simulink model "flexcan_encrypted_slave_s32k14x"  (Simulink 9.0)
settings: Solver=FixedStepDiscrete  StartTime=0.0  StopTime=10.0  FixedStep=0.1  RelTol=1e-3  EnableMultiTasking=on
PreLoadFcn:
  | mbd_s32k_examples_preload_cbk;
InitFcn:
  | mbd_s32k_consistency_checks(bdroot(gcs));
undefined symbols (not defined in the file): LQFP, Request, slave_receive_can_data, slave_send_can_data
libraries: mbd_s32k1xx_ec_toolbox x41, simulink x4
Description:
  | This model shows the usage of the FlexCAN module configured to use Flexible Data Rate and the CSEc module from the S32K14x MCUs.
  | 
  | The application will wait for frames to be received on the configured message buffer or for an event raised by pressing one of the two buttons, SW2 and SW3, which will trigger a frame send to the recipient.
  | On button SW3, the recipient toggles Red LED.
  | On button SW2, the recipient toggles Green LED.
  | 
  | The frames are sent in plain text by default, but the encrypted mode can be enabled by holding one of the buttons pressed and pressing the other.
  | The Blue LED is turned on when the encrypted mode is selected.
  | 
  | Use both maser and slave models.
  | 
  | For running the encrypted communication:
  |     The encryption uses the first non-volatile user key (KEY_1), which needs to be configured by running the CSEc Key Configuration example model (csec_keyconfig_s32k14.mdl).
  | 
  | HW prerequisite:
  | - S32K142EVB-Q100 / S32K144EVB-Q100 / S32K146EVB-Q144 / S32K148EVB-Q144
  | - Make sure that J107 has pin 1 and 2 connected and external power supply is provieded through J16.
  | 
  | Validation:
  | - The CAN Baudrate is set to 500 Kb/s.
  | - Any CAN analizer (USB to CAN device) can be used to observe CAN traffic via board CAN port J13.
PostSaveFcn:
  | mbd_s32k_examples_postsave_cbk;
settings Model: Creator=NXP MBDT Team  LastModifiedBy=nxf35172
settings DataIOCC: ExternalInput=off  InitialState=off  LimitDataPoints=on  SaveOutput=off  SignalLogging=off  SaveTime=off
settings OptimizationCC: DefaultParameterBehavior=Inlined  LifeSpan=1
settings DebuggingCC: SolverPrmCheckMsg=warning  InheritedTsInSrcMsg=none  SingleTaskRateTransMsg=error  UnconnectedInputMsg=error  UnconnectedOutputMsg=error  UnconnectedLineMsg=error  AllowSymbolicDim=off  UnknownTsInhSupMsg=error  StateNameClashWarn=warning
settings HardwareCC: ProdLargestAtomicInteger=Long  ProdLargestAtomicFloat=Double  ProdEndianess=LittleEndian  ProdHWDeviceType=ARM Compatible->ARM Cortex
settings SFSimCC: MATLABDynamicMemAlloc=off
settings RTWCC: SystemTargetFile=mbd_s32k.tlc  MakeCommand=mbd_s32k_make_rtw COPY_MDLREF_INCLUDES=0  TemplateMakefile=mbd_s32k.tmf  Description=Model Based Design Toolbox S32K14x Code Generation Target
settings CodeAppCC: IgnoreCustomStorageClasses=off
settings STFCustomTargetCC: CombineOutputUpdateFcns=on  ERTCustomFileBanners=on  SupportContinuousTime=off  SupportNonInlinedSFcns=off  RemoveResetFunc=on  MATLABClassNameForMDSCustomization=Simulink.SoftwareTarget.ERTCustomization  GRTInterface=off  SystemTargetFile=mbd_s32k14.tlc
settings ERTTargetCC: MultiwordLength=2048  ParMdlRefBuildCompliant=off  CompOptLevelCompliant=off  ConcurrentExecutionCompliant=off  ModelStepFunctionPrototypeControlCompliant=off  CPPClassGenCompliant=off  UseToolchainInfoCompliant=off  InlinedParameterPlacement=NonHierarchical  ERTCustomFileTemplate=example_file_process.tlc  ConvertIfToSwitch=off  SuppressUnreachableDefaultCases=off

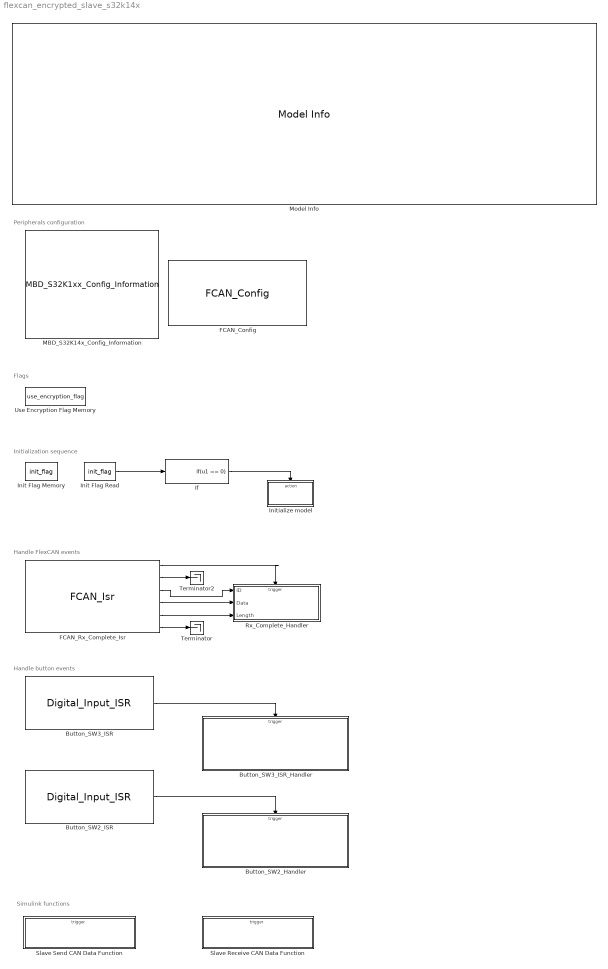
== system flexcan_encrypted_slave_s32k14x ==
  note: Simulink functions
  note: Flags
  note: Handle button events
  note: Peripherals configuration
  note: Handle FlexCAN events
  note: Initialization sequence
  "Button_SW2_Handler  " : Subsystem
  Button_SW2_ISR : mbd_s32k1xx_ec_toolbox/GPIO Blocks/Digital_Input_ISR  gpio_pin=PTC12: [PTC12 | Port C I/O]  irqc=on rising-edge  prio=15
  Button_SW3_ISR : mbd_s32k1xx_ec_toolbox/GPIO Blocks/Digital_Input_ISR  gpio_pin=PTC13: [PTC13 | Port C I/O]  irqc=on rising-edge  prio=15
  Button_SW3_ISR_Handler : Subsystem
  FCAN_Config : mbd_s32k1xx_ec_toolbox/Communication Blocks/CAN Blocks/FCAN_Config  Priority=1  can_instance=0  can_mode=Normal mode  can_max_num_mb=16  can_rx=PTE4: [CAN0_RX | CAN Rx channel]  can_tx=PTE5: [CAN0_TX | CAN Tx Channel]  show_adv_opts=on  can_clk_src=Peripheral clock  bitrate=500  bitrate_adv_opts=off  can_presdiv=7  can_rjw=3  can_pseg1=6  can_pseg2=3  can_propseg=7  can_cbt_presdiv=3  can_cbt_rjw=3  can_cbt_pseg1=5  can_cbt_pseg2=5  can_cbt_propseg=27  can_fd_enable=on  can_payload=8  can_rxfifo_enable=off  can_fifo_id_filter_extended=off  can_fifo_id_filter_remote=off  can_num_id_filters=8  can_fifo_id_format=A  can_fifo_id_filter={'0x0', '0x0', '0x0', '0x0', '0x0', '0x0', '0x0', '0x0'}  can_pn_enable=off  can_wakeup_match=off  can_wakeup_timeout=off  can_timeout_en=off  can_match_timeout=1  can_multiple_matches_en=off  can_num_matches=1  can_idfilter_extendedid=off  can_idfilter_remoteframe=off  can_idfilter_type=Match exact  can_idfilter_id1=0  can_idfilter_id2=0  can_payloadfilter_enable=on  can_payloadfilter_dlclow=0  can_payloadfilter_dlchigh=0  can_payloadfilter_type=Match exact  can_payloadfilter_payload1_b0=0  can_payloadfilter_payload1_b1=0  can_payloadfilter_payload1_b2=0  can_payloadfilter_payload1_b3=0  can_payloadfilter_payload1_b4=0  can_payloadfilter_payload1_b5=0  can_payloadfilter_payload1_b6=0  can_payloadfilter_payload1_b7=0  can_payloadfilter_payload2_b0=0  can_payloadfilter_payload2_b1=0  can_payloadfilter_payload2_b2=0  can_payloadfilter_payload2_b3=0  can_payloadfilter_payload2_b4=0  can_payloadfilter_payload2_b5=0  can_payloadfilter_payload2_b6=0  can_payloadfilter_payload2_b7=0
  FCAN_Rx_Complete_Isr : mbd_s32k1xx_ec_toolbox/Communication Blocks/CAN Blocks/FCAN_Isr  can_instance=0  can_event=Rx Complete
  If : If  IfExpression=u1 == 0  ShowElse=off
  Init Flag Memory : DataStoreMemory  DataStoreName=init_flag  ReadBeforeWriteMsg=warning  WriteAfterWriteMsg=warning  WriteAfterReadMsg=warning  ShowAdditionalParam=off  OutDataTypeStr=uint32
  Init Flag Read : DataStoreRead  DataStoreName=init_flag
  Initialize model : Subsystem  TreatAsAtomicUnit=on
  MBD_S32K14x_Config_Information : mbd_s32k1xx_ec_toolbox/MBD_S32K1xx_Config_Information  mbdt_ver=0  disp_str=|  config_params=[]  mcu_target_name=S32K144  mcu_target_package=100-LQFP  mcu_target_sram_size=64KB  mcu_system_clock_freq=80  mcu_xtal_freq=External 8  mcu_steptick_timer=LPIT Channel 0  mcu_steptick_prio=15  ds_import_enable=on  target_compiler=GCC  target_memory=FLASH  gcc_target_compile_opts=-mcpu=cortex-m4 -mthumb -mfloat-abi=hard -mfpu=fpv4-sp-d16 -O1 -g -gstrict-dwarf  gcc_target_assemble_opts=-mcpu=cortex-m4 -mthumb -mfloat-abi=hard -mfpu=fpv4-sp-d16 -g  gcc_target_link_opts=-mcpu=cortex-m4 -mthumb -mfloat-abi=hard -mfpu=fpv4-sp-d16  gcc_target_default_lcf=on  gcc_target_user_lcf=S32K144_64_flash.ld  ghs_target_compile_opts=-cpu=cortexm4f -thumb -DARM_MATH_CM4 -fpu=vfpv4_d16 -fsingle -Ogeneral -Wundef -Wimplicit-int -Wshadow -Wtrigraphs --no_commons --gnu_asm -gnu99 -gdwarf-2 -G  ghs_target_assemble_opts=-cpu=cortexm4f -fpu=vfpv4_d16  ghs_target_link_opts=-cpu=cortexm4f -thumb -fpu=vfpv4_d16  ghs_target_default_lcf=off  ghs_target_user_lcf=S32K144_64_flash.ld  iar_target_compile_opts=--cpu=Cortex-M4F --thumb --fpu=VFPv4_sp -Ol -e --debug --dlib_config normal  iar_target_assemble_opts=--cpu Cortex-M4F --thumb --fpu VFPv4_sp  iar_target_link_opts=--no_exceptions --vfe --inline  iar_target_default_lcf=off  iar_target_user_lcf=S32K144_64_flash.icf  pil_download_enable=off  rbl_download_enable=off  rbl_start_delay=5000000  rbl_download_interface=OpenSDA  rbl_restart_request=off  rbl_com_port=Custom  rbl_com_port_custom=COM1  pil_download_rate=57600  pil_opensda_drive=Custom  pil_opensda_drive_custom=D  pil_uart_instance=0  pil_uart_rx=PTA2: [LPUART0_RX | Receive]  pil_uart_tx=PTA3: [LPUART0_TX | Transmit]  FTM_PWM_PcrCheckEnDis=on  FTM_Input_Edge_Inputs_PcrCheckEnDis=on  FTM_Dual_Edge_Inputs_PcrCheckEnDis=on  FTM_Quadrature_Inputs_PcrCheckEnDis=on  FTM_Hall_Sensor_Inputs_PcrCheckEnDis=on  LPTMR_PcrCheckEnDis=on  PIT_PcrCheckEnDis=on  RTC_PcrCheckEnDis=on  FlexCAN_PcrCheckEnDis=on  LIN_PcrCheckEnDis=on  FlexIO_PcrCheckEnDis=on  LPI2C_PcrCheckEnDis=on  LPSPI_PcrCheckEnDis=on  LPUART_PcrCheckEnDis=on  CMP_PcrCheckEnDis=on  GPIO_OutputPcrCheckEnDis=on  GPIO_InputPcrCheckEnDis=on  SBC_PcrCheckEnDis=on  AMMCLIB_PcrCheckEnDis=on  FM_PcrCheckEnDis=on  Profile_PcrCheckEnDis=on  ConfigParams_PcrCheckEnDis=on  ModelRef_PcrCheckEnDis=on  PDB0_PcrCheckEnDis=on  CSEc_PcrCheckEnDis=on  eDMA_PcrCheckEnDis=on  ADC_PcrCheckEnDis=on  WDOG_PcrCheckEnDis=on
      | Target : S32K144-64KB_SRAM
      | Package : 100-pin
      | System clock : 80 MHz
      | XTAL clock : External 8 MHz
      | Compiler : GCC
      | Target Type : FLASH
      | Download Code after build : (COM1, 57600)
      | Step Tick Interrupt Priority : 15
  Model Info : simulink/Model-Wide Utilities/Model Info  Frame=on  DisplayStringWithTags=|  HorizontalTextAlignment=Left  LeftAlignmentValue=0.02
      | Model Name: %<ModelName>
      | 
      | Description: %<Description>
  Rx_Complete_Handler : Subsystem  TreatAsAtomicUnit=on
      settings: RTWSystemCode=Nonreusable function
  Slave Receive CAN Data Function : Subsystem  TreatAsAtomicUnit=on
  Slave Send CAN Data Function : Subsystem  TreatAsAtomicUnit=on
  Terminator : Terminator
  Terminator2 : Terminator
  Use Encryption Flag Memory : DataStoreMemory  DataStoreName=use_encryption_flag  ReadBeforeWriteMsg=warning  WriteAfterWriteMsg=warning  WriteAfterReadMsg=warning  ShowAdditionalParam=off
  wires:
  If/1 -> Initialize model/Action
  Init Flag Read/1 -> If/1
  FCAN_Rx_Complete_Isr/1 -> Rx_Complete_Handler/Trigger
  FCAN_Rx_Complete_Isr/3 -> Rx_Complete_Handler/1(ID)
  FCAN_Rx_Complete_Isr/2 -> Terminator2/1
  Button_SW3_ISR/1 -> Button_SW3_ISR_Handler/Trigger
  Button_SW2_ISR/1 -> "Button_SW2_Handler  "/Trigger
  FCAN_Rx_Complete_Isr/4 -> Rx_Complete_Handler/2(Data)
  FCAN_Rx_Complete_Isr/6 -> Terminator/1
  FCAN_Rx_Complete_Isr/5 -> Rx_Complete_Handler/3(Length)

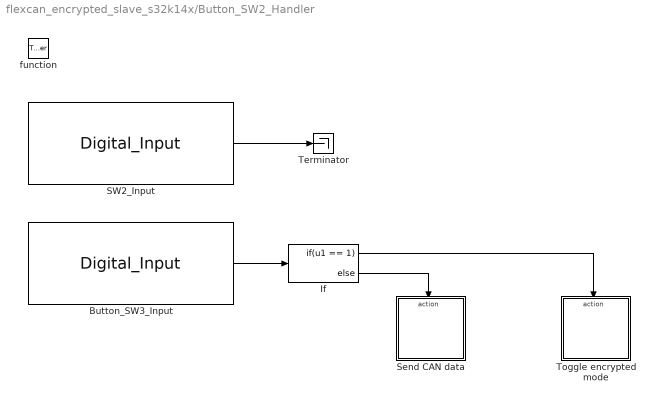
== system flexcan_encrypted_slave_s32k14x/Button_SW2_Handler   ==
  function : TriggerPort  TriggerType=function-call  VariantControl=Variant
  Button_SW3_Input : mbd_s32k1xx_ec_toolbox/GPIO Blocks/Digital_Input  gpio_pin=PTC13: [PTC13 | Port C I/O]  pull_resistor=None  passive_filter=off
  If : If  IfExpression=u1 == 1
  SW2_Input : mbd_s32k1xx_ec_toolbox/GPIO Blocks/Digital_Input  gpio_pin=PTC12: [PTC12 | Port C I/O]  pull_resistor=None  passive_filter=off
  Send CAN data : Subsystem
  Terminator : Terminator
  Toggle encrypted mode : Subsystem
  wires:
  SW2_Input/1 -> Terminator/1
  If/2 -> Send CAN data/Action
  If/1 -> Toggle encrypted mode/Action
  Button_SW3_Input/1 -> If/1

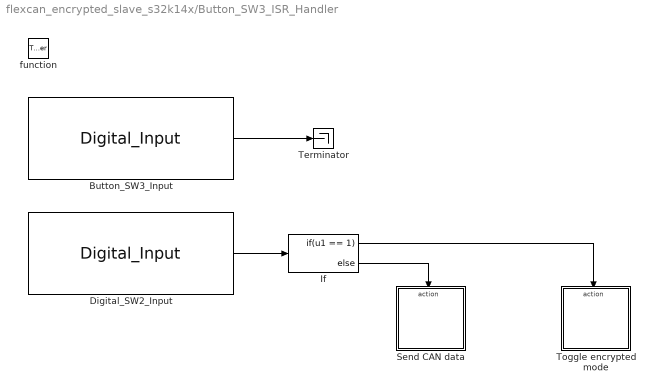
== system flexcan_encrypted_slave_s32k14x/Button_SW3_ISR_Handler ==
  function : TriggerPort  TriggerType=function-call  VariantControl=Variant
  Button_SW3_Input : mbd_s32k1xx_ec_toolbox/GPIO Blocks/Digital_Input  gpio_pin=PTC13: [PTC13 | Port C I/O]  pull_resistor=None  passive_filter=off
  Digital_SW2_Input : mbd_s32k1xx_ec_toolbox/GPIO Blocks/Digital_Input  gpio_pin=PTC12: [PTC12 | Port C I/O]  pull_resistor=None  passive_filter=off
  If : If  IfExpression=u1 == 1
  Send CAN data : Subsystem
  Terminator : Terminator
  Toggle encrypted mode : Subsystem
  wires:
  If/2 -> Send CAN data/Action
  If/1 -> Toggle encrypted mode/Action
  Digital_SW2_Input/1 -> If/1
  Button_SW3_Input/1 -> Terminator/1

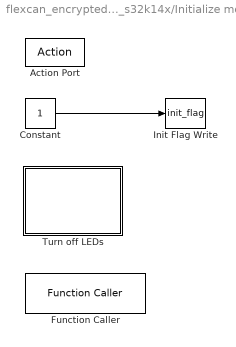
== system flexcan_encrypted_slave_s32k14x/Initialize model ==
  Action Port : ActionPort
  Constant : Constant  OutDataTypeStr=uint32
  Function Caller : FunctionCaller  Priority=2  FunctionPrototype=slave_receive_can_data()
  Init Flag Write : DataStoreWrite  DataStoreName=init_flag
  Turn off LEDs : Subsystem  Priority=1
  wires:
  Constant/1 -> Init Flag Write/1

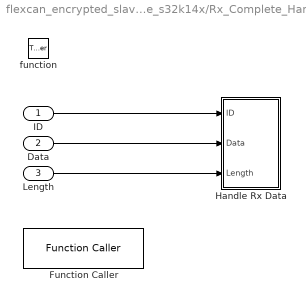
== system flexcan_encrypted_slave_s32k14x/Rx_Complete_Handler ==
  ID : Inport
  Data : Inport  Port=2
  Length : Inport  Port=3
  function : TriggerPort  TriggerType=function-call  VariantControl=Variant
  Function Caller : FunctionCaller  Priority=2  FunctionPrototype=slave_receive_can_data()
  Handle Rx Data : Subsystem  Priority=1
  wires:
  ID/1 -> Handle Rx Data/1(ID)
  Data/1 -> Handle Rx Data/2(Data)
  Length/1 -> Handle Rx Data/3(Length)

== system flexcan_encrypted_slave_s32k14x/Slave Receive CAN Data Function ==
  slave_receive_can_data : TriggerPort  TriggerType=function-call  IsSimulinkFunction=on  FunctionName=slave_receive_can_data  VariantControl=Variant
  FCAN_Receive_ID_0x2 : mbd_s32k1xx_ec_toolbox/Communication Blocks/CAN Blocks/FCAN_Receive  can_instance=0  can_mode=Non-blocking  can_timeout_ms=0  can_mb_idx=1  can_extended_id=off  can_is_remote=off  can_id=1  can_msg_mask=FFFFFFFF  show_adv_opts=on  can_use_rxfifo=off  can_fd_enable=on

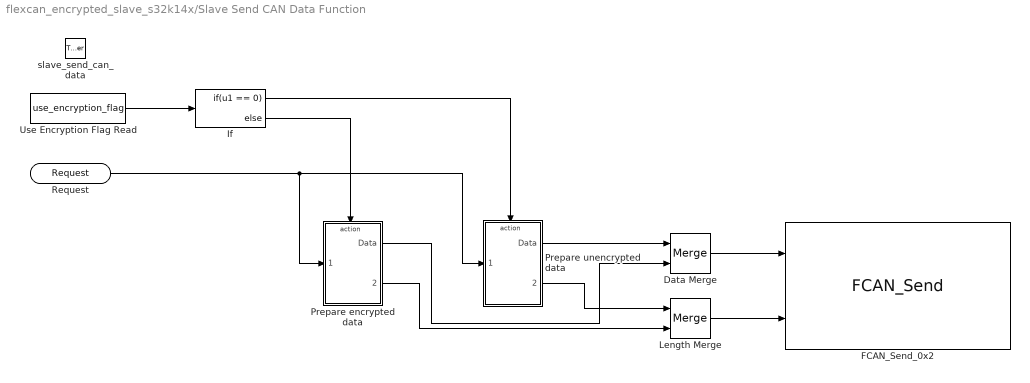
== system flexcan_encrypted_slave_s32k14x/Slave Send CAN Data Function ==
  slave_send_can_data : TriggerPort  TriggerType=function-call  IsSimulinkFunction=on  FunctionName=slave_send_can_data  VariantControl=Variant
  Data Merge : Merge  AllowUnequalInputPortWidths=on
  FCAN_Send_0x2 : mbd_s32k1xx_ec_toolbox/Communication Blocks/CAN Blocks/FCAN_Send  can_instance=0  can_mode=Non-blocking  can_timeout_ms=0  can_mb_idx=0  can_extended_id=off  can_is_remote=off  can_id=2  show_adv_opts=on  can_fd_enable=on  can_enable_brs=on  can_fd_padding=0
  If : If  IfExpression=u1 == 0
  Length Merge : Merge
  Prepare encrypted data : Subsystem
  Prepare unencrypted data : Subsystem
  Use Encryption Flag Read : DataStoreRead  DataStoreName=use_encryption_flag
  Request : ArgIn  DisableCoverage=on  OutDataTypeStr=uint8  ArgumentName=Request
  wires:
  Use Encryption Flag Read/1 -> If/1
  If/2 -> Prepare encrypted data/Action
  If/1 -> Prepare unencrypted data/Action
  Prepare unencrypted data/1(Data) -> Data Merge/1
  Prepare encrypted data/1(Data) -> Data Merge/2
  Prepare unencrypted data/2(Length) -> Length Merge/1
  Prepare encrypted data/2(Length) -> Length Merge/2
  Data Merge/1 -> FCAN_Send_0x2/1
  Length Merge/1 -> FCAN_Send_0x2/2
  Request/1 -> Prepare encrypted data/1(Request), Prepare unencrypted data/1(Request)

== system flexcan_encrypted_slave_s32k14x/Button_SW2_Handler  /Send CAN data ==
  Action Port : ActionPort
  Constant : Constant  OutDataTypeStr=uint8
  Function Caller : FunctionCaller  FunctionPrototype=slave_send_can_data(Request)  InputArgumentSpecifications=uint8(1)
  wires:
  Constant/1 -> Function Caller/1

== system flexcan_encrypted_slave_s32k14x/Button_SW2_Handler  /Toggle encrypted mode ==
  Action Port : ActionPort
  Blue LED : Subsystem  Variant=on
      mask Display:
      | disp('Blue LED');
      | port_label('input',1,'out')
  Logical Operator : Logic  Operator=NOT  AllPortsSameDT=off  OutDataTypeStr=boolean
  Use Encryption Flag Read : DataStoreRead  DataStoreName=use_encryption_flag
  Use Encryption Flag Write : DataStoreWrite  DataStoreName=use_encryption_flag
  wires:
  Use Encryption Flag Read/1 -> Logical Operator/1
  Logical Operator/1 -> Blue LED/1(In1), Use Encryption Flag Write/1

== system flexcan_encrypted_slave_s32k14x/Button_SW3_ISR_Handler/Send CAN data ==
  Action Port : ActionPort
  Constant : Constant  Value=0  OutDataTypeStr=uint8
  Function Caller : FunctionCaller  FunctionPrototype=slave_send_can_data(Request)  InputArgumentSpecifications=uint8(1)
  wires:
  Constant/1 -> Function Caller/1

== system flexcan_encrypted_slave_s32k14x/Button_SW3_ISR_Handler/Toggle encrypted mode ==
  Action Port : ActionPort
  Blue LED : Subsystem  Variant=on
      mask Display:
      | disp('Blue LED');
      | port_label('input',1,'out')
  Logical Operator : Logic  Operator=NOT  AllPortsSameDT=off  OutDataTypeStr=boolean
  Use Encryption Flag Read : DataStoreRead  DataStoreName=use_encryption_flag
  Use Encryption Flag Write : DataStoreWrite  DataStoreName=use_encryption_flag
  wires:
  Use Encryption Flag Read/1 -> Logical Operator/1
  Logical Operator/1 -> Blue LED/1(In1), Use Encryption Flag Write/1

== system flexcan_encrypted_slave_s32k14x/Initialize model/Turn off LEDs ==
  Blue LED off : Subsystem
      mask Display: disp('Blue LED off');
  Green LED off : Subsystem
      mask Display: disp('Green LED off');
  Red LED off : Subsystem
      mask Display: disp('Red LED off');

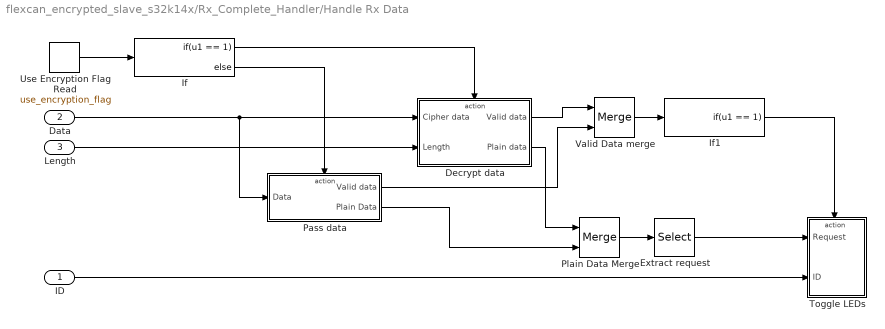
== system flexcan_encrypted_slave_s32k14x/Rx_Complete_Handler/Handle Rx Data ==
  ID : Inport
  Data : Inport  Port=2
  Length : Inport  Port=3
  Decrypt data : Subsystem  TreatAsAtomicUnit=on
  Extract request : Selector  IndexOptions=Index vector (dialog)  Indices=[1]  OutputSizes=1
  If : If  IfExpression=u1 == 1
  If1 : If  IfExpression=u1 == 1  ShowElse=off
  Pass data : Subsystem  TreatAsAtomicUnit=on
  Plain Data Merge : Merge  AllowUnequalInputPortWidths=on
  Toggle LEDs : Subsystem
  Use Encryption Flag Read : DataStoreRead  DataStoreName=use_encryption_flag
  Valid Data merge : Merge  AllowUnequalInputPortWidths=on
  wires:
  If1/1 -> Toggle LEDs/Action
  Data/1 -> Pass data/1(Data), Decrypt data/1(Cipher data)
  Use Encryption Flag Read/1 -> If/1
  If/1 -> Decrypt data/Action
  Plain Data Merge/1 -> Extract request/1
  Decrypt data/2(Plain data) -> Plain Data Merge/1
  Extract request/1 -> Toggle LEDs/1(Request)
  ID/1 -> Toggle LEDs/2(ID)
  Pass data/2(Plain Data) -> Plain Data Merge/2
  If/2 -> Pass data/Action
  Length/1 -> Decrypt data/2(Length)
  Decrypt data/1(Valid data) -> Valid Data merge/1
  Valid Data merge/1 -> If1/1
  Pass data/1(Valid data) -> Valid Data merge/2

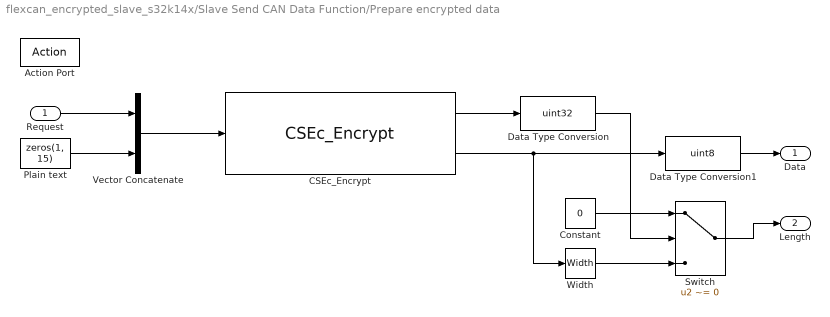
== system flexcan_encrypted_slave_s32k14x/Slave Send CAN Data Function/Prepare encrypted data ==
  Request : Inport
  Action Port : ActionPort
  CSEc_Encrypt : mbd_s32k1xx_ec_toolbox/Core and System Blocks/CSEc Blocks/CSEc_Encrypt  Priority=2  csec_mode=Electronic Codebook (ECB)  csec_key_id=KEY_1  csec_timeout=1
  Constant : Constant  Value=0  OutDataTypeStr=uint8
  Data Type Conversion : DataTypeConversion  OutDataTypeStr=uint32
  Data Type Conversion1 : DataTypeConversion  OutDataTypeStr=uint8
  Plain text : Constant  Value=zeros(1, 15)  OutDataTypeStr=uint8
  Switch : Switch  Criteria=u2 ~= 0
  Vector Concatenate : Concatenate  Priority=1
  Width : Width  DataType=uint8
  Data : Outport
  Length : Outport  Port=2
  wires:
  CSEc_Encrypt/1 -> Data Type Conversion/1
  CSEc_Encrypt/2 -> Width/1, Data Type Conversion1/1
  Vector Concatenate/1 -> CSEc_Encrypt/1
  Plain text/1 -> Vector Concatenate/2
  Request/1 -> Vector Concatenate/1
  Data Type Conversion/1 -> Switch/2
  Width/1 -> Switch/3
  Switch/1 -> Length/1
  Data Type Conversion1/1 -> Data/1
  Constant/1 -> Switch/1

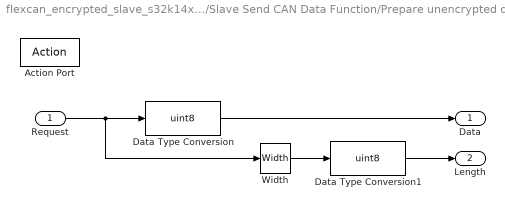
== system flexcan_encrypted_slave_s32k14x/Slave Send CAN Data Function/Prepare unencrypted data ==
  Request : Inport
  Action Port : ActionPort
  Data Type Conversion : DataTypeConversion  OutDataTypeStr=uint8
  Data Type Conversion1 : DataTypeConversion  OutDataTypeStr=uint8
  Width : Width  DataType=uint8
  Data : Outport
  Length : Outport  Port=2
  wires:
  Request/1 -> Width/1, Data Type Conversion/1
  Data Type Conversion/1 -> Data/1
  Data Type Conversion1/1 -> Length/1
  Width/1 -> Data Type Conversion1/1

== system flexcan_encrypted_slave_s32k14x/Button_SW2_Handler  /Toggle encrypted mode/Blue LED ==
  note: 1) Add Subsystem or Model blocks as valid variant choices.
      | 2) You cannot connect blocks at this level. At simulation, connectivity is automatically
      | determined, based on the active variant and port name matching.
  In1 : Inport
  S32K142 : Subsystem  VariantControl=VSS_S32k142
  S32K144 : Subsystem  VariantControl=VSS_S32k144
  S32K146 : Subsystem  VariantControl=VSS_S32k146
  S32K148 : Subsystem  VariantControl=VSS_S32k148

== system flexcan_encrypted_slave_s32k14x/Button_SW3_ISR_Handler/Toggle encrypted mode/Blue LED ==
  note: 1) Add Subsystem or Model blocks as valid variant choices.
      | 2) You cannot connect blocks at this level. At simulation, connectivity is automatically
      | determined, based on the active variant and port name matching.
  In1 : Inport
  S32K142 : Subsystem  VariantControl=VSS_S32k142
  S32K144 : Subsystem  VariantControl=VSS_S32k144
  S32K146 : Subsystem  VariantControl=VSS_S32k146
  S32K148 : Subsystem  VariantControl=VSS_S32k148

== system flexcan_encrypted_slave_s32k14x/Initialize model/Turn off LEDs/Blue LED off ==
  Blue LED : Subsystem  Variant=on
      mask Display:
      | disp('Blue LED');
      | port_label('input',1,'out')
  Constant : Constant  Value=0  OutDataTypeStr=boolean
  wires:
  Constant/1 -> Blue LED/1(In1)

== system flexcan_encrypted_slave_s32k14x/Initialize model/Turn off LEDs/Green LED off ==
  Constant : Constant  Value=0  OutDataTypeStr=boolean
  Green LED : Subsystem  Variant=on
      mask Display:
      | disp('Green LED');
      | port_label('input',1,'out')
  wires:
  Constant/1 -> Green LED/1(In1)

== system flexcan_encrypted_slave_s32k14x/Initialize model/Turn off LEDs/Red LED off ==
  Constant : Constant  Value=0  OutDataTypeStr=boolean
  Red LED : Subsystem  Variant=on
      mask Display:
      | disp('Red LED');
      | port_label('input',1,'out')
  wires:
  Constant/1 -> Red LED/1(In1)

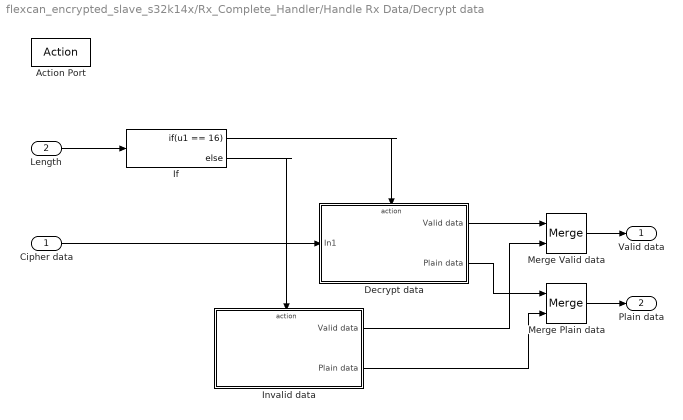
== system flexcan_encrypted_slave_s32k14x/Rx_Complete_Handler/Handle Rx Data/Decrypt data ==
  Cipher data : Inport
  Length : Inport  Port=2
  Action Port : ActionPort
  Decrypt data : Subsystem
  If : If  IfExpression=u1 == 16
  Invalid data : Subsystem
  Merge Plain data : Merge  AllowUnequalInputPortWidths=on
  Merge Valid data : Merge
  Valid data : Outport
  Plain data : Outport  Port=2
  wires:
  Length/1 -> If/1
  Cipher data/1 -> Decrypt data/1(In1)
  If/1 -> Decrypt data/Action
  If/2 -> Invalid data/Action
  Merge Valid data/1 -> Valid data/1
  Decrypt data/1(Valid data) -> Merge Valid data/1
  Invalid data/1(Valid data) -> Merge Valid data/2
  Merge Plain data/1 -> Plain data/1
  Decrypt data/2(Plain data) -> Merge Plain data/1
  Invalid data/2(Plain data) -> Merge Plain data/2

== system flexcan_encrypted_slave_s32k14x/Rx_Complete_Handler/Handle Rx Data/Pass data ==
  Data : Inport
  Action Port : ActionPort
  Constant : Constant  OutDataTypeStr=boolean
  Valid data : Outport  InitialOutput=1
  Plain Data : Outport  Port=2
  wires:
  Data/1 -> Plain Data/1
  Constant/1 -> Valid data/1

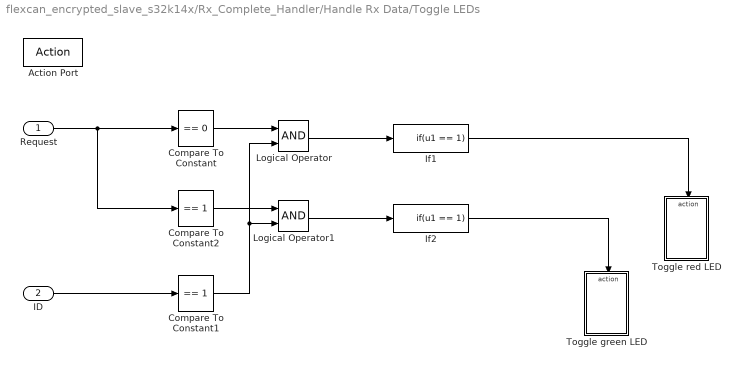
== system flexcan_encrypted_slave_s32k14x/Rx_Complete_Handler/Handle Rx Data/Toggle LEDs ==
  Request : Inport  OutDataTypeStr=uint8
  ID : Inport  Port=2
  Action Port : ActionPort
  Compare To Constant : simulink/Logic and Bit Operations/Compare To Constant  relop===  const=0  OutDataTypeStr=boolean
  Compare To Constant1 : simulink/Logic and Bit Operations/Compare To Constant  relop===  const=1  OutDataTypeStr=boolean
  Compare To Constant2 : simulink/Logic and Bit Operations/Compare To Constant  relop===  const=1  OutDataTypeStr=boolean
  If1 : If  IfExpression=u1 == 1  ShowElse=off
  If2 : If  IfExpression=u1 == 1  ShowElse=off
  Logical Operator : Logic  AllPortsSameDT=off  OutDataTypeStr=boolean
  Logical Operator1 : Logic  AllPortsSameDT=off  OutDataTypeStr=boolean
  Toggle green LED : Subsystem
  Toggle red LED : Subsystem
  wires:
  ID/1 -> Compare To Constant1/1
  Request/1 -> Compare To Constant2/1, Compare To Constant/1
  If2/1 -> Toggle green LED/Action
  If1/1 -> Toggle red LED/Action
  Compare To Constant/1 -> Logical Operator/1
  Compare To Constant1/1 -> Logical Operator/2, Logical Operator1/2
  Logical Operator/1 -> If1/1
  Compare To Constant2/1 -> Logical Operator1/1
  Logical Operator1/1 -> If2/1

== system flexcan_encrypted_slave_s32k14x/Button_SW2_Handler  /Toggle encrypted mode/Blue LED/S32K142 ==
  In1 : Inport
  Blue_LED : mbd_s32k1xx_ec_toolbox/GPIO Blocks/Digital_Output  gpio_pin=PTD0: [PTD0 | Port D I/O]  init_val=Low  drive_strength=Low
  wires:
  In1/1 -> Blue_LED/1

== system flexcan_encrypted_slave_s32k14x/Button_SW2_Handler  /Toggle encrypted mode/Blue LED/S32K144 ==
  In1 : Inport
  Blue_LED : mbd_s32k1xx_ec_toolbox/GPIO Blocks/Digital_Output  gpio_pin=PTD0: [PTD0 | Port D I/O]  init_val=Low  drive_strength=Low
  Logical Operator : Logic  Operator=NOT  AllPortsSameDT=off  OutDataTypeStr=boolean
  wires:
  In1/1 -> Logical Operator/1
  Logical Operator/1 -> Blue_LED/1

== system flexcan_encrypted_slave_s32k14x/Button_SW2_Handler  /Toggle encrypted mode/Blue LED/S32K146 ==
  In1 : Inport
  Blue_LED : mbd_s32k1xx_ec_toolbox/GPIO Blocks/Digital_Output  gpio_pin=PTD0: [PTD0 | Port D I/O]  init_val=Low  drive_strength=Low
  wires:
  In1/1 -> Blue_LED/1

== system flexcan_encrypted_slave_s32k14x/Button_SW2_Handler  /Toggle encrypted mode/Blue LED/S32K148 ==
  In1 : Inport
  Blue_LED : mbd_s32k1xx_ec_toolbox/GPIO Blocks/Digital_Output  gpio_pin=PTE23: [PTE23 | Port E I/O]  init_val=Low  drive_strength=Low
  wires:
  In1/1 -> Blue_LED/1

== system flexcan_encrypted_slave_s32k14x/Button_SW3_ISR_Handler/Toggle encrypted mode/Blue LED/S32K142 ==
  In1 : Inport
  Blue_LED : mbd_s32k1xx_ec_toolbox/GPIO Blocks/Digital_Output  gpio_pin=PTD0: [PTD0 | Port D I/O]  init_val=Low  drive_strength=Low
  wires:
  In1/1 -> Blue_LED/1

== system flexcan_encrypted_slave_s32k14x/Button_SW3_ISR_Handler/Toggle encrypted mode/Blue LED/S32K144 ==
  In1 : Inport
  Blue_LED : mbd_s32k1xx_ec_toolbox/GPIO Blocks/Digital_Output  gpio_pin=PTD0: [PTD0 | Port D I/O]  init_val=Low  drive_strength=Low
  Logical Operator : Logic  Operator=NOT  AllPortsSameDT=off  OutDataTypeStr=boolean
  wires:
  In1/1 -> Logical Operator/1
  Logical Operator/1 -> Blue_LED/1

== system flexcan_encrypted_slave_s32k14x/Button_SW3_ISR_Handler/Toggle encrypted mode/Blue LED/S32K146 ==
  In1 : Inport
  Blue_LED : mbd_s32k1xx_ec_toolbox/GPIO Blocks/Digital_Output  gpio_pin=PTD0: [PTD0 | Port D I/O]  init_val=Low  drive_strength=Low
  wires:
  In1/1 -> Blue_LED/1

== system flexcan_encrypted_slave_s32k14x/Button_SW3_ISR_Handler/Toggle encrypted mode/Blue LED/S32K148 ==
  In1 : Inport
  Blue_LED : mbd_s32k1xx_ec_toolbox/GPIO Blocks/Digital_Output  gpio_pin=PTE23: [PTE23 | Port E I/O]  init_val=Low  drive_strength=Low
  wires:
  In1/1 -> Blue_LED/1

== system flexcan_encrypted_slave_s32k14x/Initialize model/Turn off LEDs/Blue LED off/Blue LED ==
  note: 1) Add Subsystem or Model blocks as valid variant choices.
      | 2) You cannot connect blocks at this level. At simulation, connectivity is automatically
      | determined, based on the active variant and port name matching.
  In1 : Inport
  S32K142 : Subsystem  VariantControl=VSS_S32k142
  S32K144 : Subsystem  VariantControl=VSS_S32k144
  S32K146 : Subsystem  VariantControl=VSS_S32k146
  S32K148 : Subsystem  VariantControl=VSS_S32k148

== system flexcan_encrypted_slave_s32k14x/Initialize model/Turn off LEDs/Green LED off/Green LED ==
  note: 1) Add Subsystem or Model blocks as valid variant choices.
      | 2) You cannot connect blocks at this level. At simulation, connectivity is automatically
      | determined, based on the active variant and port name matching.
  In1 : Inport
  S32K142 : Subsystem  VariantControl=VSS_S32k142
  S32K144 : Subsystem  VariantControl=VSS_S32k144
  S32K146 : Subsystem  VariantControl=VSS_S32k146
  S32K148 : Subsystem  VariantControl=VSS_S32k148

== system flexcan_encrypted_slave_s32k14x/Initialize model/Turn off LEDs/Red LED off/Red LED ==
  note: 1) Add Subsystem or Model blocks as valid variant choices.
      | 2) You cannot connect blocks at this level. At simulation, connectivity is automatically
      | determined, based on the active variant and port name matching.
  In1 : Inport
  S32K142 : Subsystem  VariantControl=VSS_S32k142
  S32K144 : Subsystem  VariantControl=VSS_S32k144
  S32K146 : Subsystem  VariantControl=VSS_S32k146
  S32K148 : Subsystem  VariantControl=VSS_S32k148

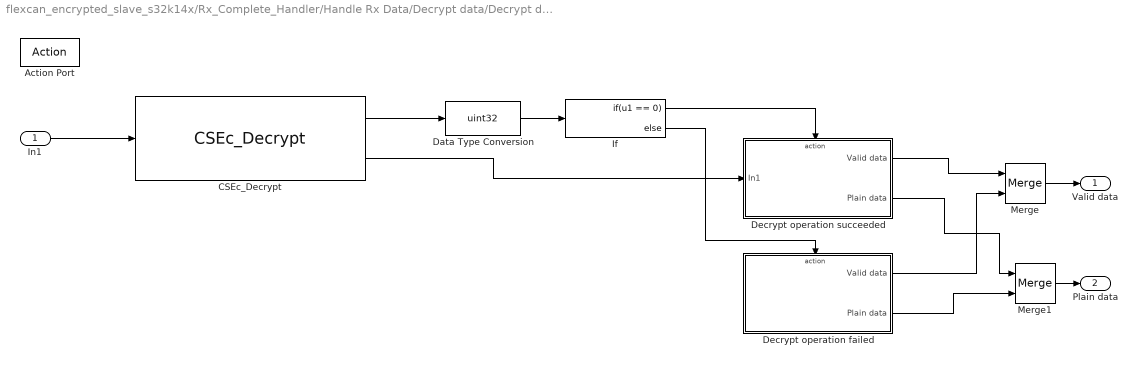
== system flexcan_encrypted_slave_s32k14x/Rx_Complete_Handler/Handle Rx Data/Decrypt data/Decrypt data ==
  In1 : Inport
  Action Port : ActionPort
  CSEc_Decrypt : mbd_s32k1xx_ec_toolbox/Core and System Blocks/CSEc Blocks/CSEc_Decrypt  csec_mode=Electronic Codebook (ECB)  csec_key_id=KEY_1  csec_timeout=1
  Data Type Conversion : DataTypeConversion  OutDataTypeStr=uint32
  Decrypt operation failed : Subsystem
  Decrypt operation succeeded : Subsystem
  If : If  IfExpression=u1 == 0
  Merge : Merge
  Merge1 : Merge  AllowUnequalInputPortWidths=on
  Valid data : Outport
  Plain data : Outport  Port=2  InitialOutput=0
  wires:
  In1/1 -> CSEc_Decrypt/1
  CSEc_Decrypt/2 -> Decrypt operation succeeded/1(In1)
  Decrypt operation succeeded/2(Plain data) -> Merge1/1
  Decrypt operation succeeded/1(Valid data) -> Merge/1
  CSEc_Decrypt/1 -> Data Type Conversion/1
  If/1 -> Decrypt operation succeeded/Action
  Decrypt operation failed/2(Plain data) -> Merge1/2
  If/2 -> Decrypt operation failed/Action
  Decrypt operation failed/1(Valid data) -> Merge/2
  Merge/1 -> Valid data/1
  Merge1/1 -> Plain data/1
  Data Type Conversion/1 -> If/1

== system flexcan_encrypted_slave_s32k14x/Rx_Complete_Handler/Handle Rx Data/Decrypt data/Invalid data ==
  Action Port : ActionPort
  Constant1 : Constant  Value=0  OutDataTypeStr=uint8
  Invalid data : Constant  Value=0  OutDataTypeStr=boolean
  Valid data : Outport  InitialOutput=0
  Plain data : Outport  Port=2  InitialOutput=0
  wires:
  Invalid data/1 -> Valid data/1
  Constant1/1 -> Plain data/1

== system flexcan_encrypted_slave_s32k14x/Rx_Complete_Handler/Handle Rx Data/Toggle LEDs/Toggle green LED ==
  Action Port : ActionPort
  Chart : Stateflow chart  TreatAsAtomicUnit=on
  Green LED : Subsystem  Variant=on
      mask Display:
      | disp('Green LED');
      | port_label('input',1,'out')
  wires:
  Chart/1(" A") -> Green LED/1(In1)

== system flexcan_encrypted_slave_s32k14x/Rx_Complete_Handler/Handle Rx Data/Toggle LEDs/Toggle red LED ==
  Action Port : ActionPort
  Chart : Stateflow chart  TreatAsAtomicUnit=on
  Red LED : Subsystem  Variant=on
      mask Display:
      | disp('Red LED');
      | port_label('input',1,'out')
  wires:
  Chart/1(" A") -> Red LED/1(In1)

== system flexcan_encrypted_slave_s32k14x/Initialize model/Turn off LEDs/Blue LED off/Blue LED/S32K142 ==
  In1 : Inport
  Blue_LED : mbd_s32k1xx_ec_toolbox/GPIO Blocks/Digital_Output  gpio_pin=PTD0: [PTD0 | Port D I/O]  init_val=Low  drive_strength=Low
  wires:
  In1/1 -> Blue_LED/1

== system flexcan_encrypted_slave_s32k14x/Initialize model/Turn off LEDs/Blue LED off/Blue LED/S32K144 ==
  In1 : Inport
  Blue_LED : mbd_s32k1xx_ec_toolbox/GPIO Blocks/Digital_Output  gpio_pin=PTD0: [PTD0 | Port D I/O]  init_val=Low  drive_strength=Low
  Logical Operator : Logic  Operator=NOT  AllPortsSameDT=off  OutDataTypeStr=boolean
  wires:
  In1/1 -> Logical Operator/1
  Logical Operator/1 -> Blue_LED/1

== system flexcan_encrypted_slave_s32k14x/Initialize model/Turn off LEDs/Blue LED off/Blue LED/S32K146 ==
  In1 : Inport
  Blue_LED : mbd_s32k1xx_ec_toolbox/GPIO Blocks/Digital_Output  gpio_pin=PTD0: [PTD0 | Port D I/O]  init_val=Low  drive_strength=Low
  wires:
  In1/1 -> Blue_LED/1

== system flexcan_encrypted_slave_s32k14x/Initialize model/Turn off LEDs/Blue LED off/Blue LED/S32K148 ==
  In1 : Inport
  Blue_LED : mbd_s32k1xx_ec_toolbox/GPIO Blocks/Digital_Output  gpio_pin=PTE23: [PTE23 | Port E I/O]  init_val=Low  drive_strength=Low
  wires:
  In1/1 -> Blue_LED/1

== system flexcan_encrypted_slave_s32k14x/Initialize model/Turn off LEDs/Green LED off/Green LED/S32K142 ==
  In1 : Inport
  Green_LED : mbd_s32k1xx_ec_toolbox/GPIO Blocks/Digital_Output  gpio_pin=PTD16: [PTD16 | Port D I/O]  init_val=Low  drive_strength=Low
  wires:
  In1/1 -> Green_LED/1

== system flexcan_encrypted_slave_s32k14x/Initialize model/Turn off LEDs/Green LED off/Green LED/S32K144 ==
  In1 : Inport
  Green_LED : mbd_s32k1xx_ec_toolbox/GPIO Blocks/Digital_Output  gpio_pin=PTD16: [PTD16 | Port D I/O]  init_val=Low  drive_strength=Low
  Logical Operator : Logic  Operator=NOT  AllPortsSameDT=off  OutDataTypeStr=boolean
  wires:
  In1/1 -> Logical Operator/1
  Logical Operator/1 -> Green_LED/1

== system flexcan_encrypted_slave_s32k14x/Initialize model/Turn off LEDs/Green LED off/Green LED/S32K146 ==
  In1 : Inport
  Green_LED : mbd_s32k1xx_ec_toolbox/GPIO Blocks/Digital_Output  gpio_pin=PTD16: [PTD16 | Port D I/O]  init_val=Low  drive_strength=Low
  wires:
  In1/1 -> Green_LED/1

== system flexcan_encrypted_slave_s32k14x/Initialize model/Turn off LEDs/Green LED off/Green LED/S32K148 ==
  In1 : Inport
  Green_LED : mbd_s32k1xx_ec_toolbox/GPIO Blocks/Digital_Output  gpio_pin=PTE22: [PTE22 | Port E I/O]  init_val=Low  drive_strength=Low
  wires:
  In1/1 -> Green_LED/1

== system flexcan_encrypted_slave_s32k14x/Initialize model/Turn off LEDs/Red LED off/Red LED/S32K142 ==
  In1 : Inport
  Red_LED : mbd_s32k1xx_ec_toolbox/GPIO Blocks/Digital_Output  gpio_pin=PTD15: [PTD15 | Port D I/O]  init_val=Low  drive_strength=Low
  wires:
  In1/1 -> Red_LED/1

== system flexcan_encrypted_slave_s32k14x/Initialize model/Turn off LEDs/Red LED off/Red LED/S32K144 ==
  In1 : Inport
  Logical Operator : Logic  Operator=NOT  AllPortsSameDT=off  OutDataTypeStr=boolean
  Red_LED : mbd_s32k1xx_ec_toolbox/GPIO Blocks/Digital_Output  gpio_pin=PTD15: [PTD15 | Port D I/O]  init_val=Low  drive_strength=Low
  wires:
  In1/1 -> Logical Operator/1
  Logical Operator/1 -> Red_LED/1

== system flexcan_encrypted_slave_s32k14x/Initialize model/Turn off LEDs/Red LED off/Red LED/S32K146 ==
  In1 : Inport
  Red_LED : mbd_s32k1xx_ec_toolbox/GPIO Blocks/Digital_Output  gpio_pin=PTD15: [PTD15 | Port D I/O]  init_val=Low  drive_strength=Low
  wires:
  In1/1 -> Red_LED/1

== system flexcan_encrypted_slave_s32k14x/Initialize model/Turn off LEDs/Red LED off/Red LED/S32K148 ==
  In1 : Inport
  Red_LED : mbd_s32k1xx_ec_toolbox/GPIO Blocks/Digital_Output  gpio_pin=PTE21: [PTE21 | Port E I/O]  init_val=Low  drive_strength=Low
  wires:
  In1/1 -> Red_LED/1

== system flexcan_encrypted_slave_s32k14x/Rx_Complete_Handler/Handle Rx Data/Decrypt data/Decrypt data/Decrypt operation failed ==
  Action Port : ActionPort
  Constant : Constant  Value=0  OutDataTypeStr=uint8
  Invalid data : Constant  OutDataTypeStr=boolean
  Valid data : Outport  InitialOutput=0
  Plain data : Outport  Port=2  InitialOutput=0
  wires:
  Invalid data/1 -> Valid data/1
  Constant/1 -> Plain data/1

== system flexcan_encrypted_slave_s32k14x/Rx_Complete_Handler/Handle Rx Data/Decrypt data/Decrypt data/Decrypt operation succeeded ==
  In1 : Inport
  Action Port : ActionPort
  Invalid data : Constant  OutDataTypeStr=boolean
  Valid data : Outport  InitialOutput=0
  Plain data : Outport  Port=2
  wires:
  Invalid data/1 -> Valid data/1
  In1/1 -> Plain data/1

== system flexcan_encrypted_slave_s32k14x/Rx_Complete_Handler/Handle Rx Data/Toggle LEDs/Toggle green LED/Green LED ==
  note: 1) Add Subsystem or Model blocks as valid variant choices.
      | 2) You cannot connect blocks at this level. At simulation, connectivity is automatically
      | determined, based on the active variant and port name matching.
  In1 : Inport
  S32K142 : Subsystem  VariantControl=VSS_S32k142
  S32K144 : Subsystem  VariantControl=VSS_S32k144
  S32K146 : Subsystem  VariantControl=VSS_S32k146
  S32K148 : Subsystem  VariantControl=VSS_S32k148

== system flexcan_encrypted_slave_s32k14x/Rx_Complete_Handler/Handle Rx Data/Toggle LEDs/Toggle red LED/Red LED ==
  note: 1) Add Subsystem or Model blocks as valid variant choices.
      | 2) You cannot connect blocks at this level. At simulation, connectivity is automatically
      | determined, based on the active variant and port name matching.
  In1 : Inport
  S32K142 : Subsystem  VariantControl=VSS_S32k142
  S32K144 : Subsystem  VariantControl=VSS_S32k144
  S32K146 : Subsystem  VariantControl=VSS_S32k146
  S32K148 : Subsystem  VariantControl=VSS_S32k148

== system flexcan_encrypted_slave_s32k14x/Rx_Complete_Handler/Handle Rx Data/Toggle LEDs/Toggle green LED/Green LED/S32K142 ==
  In1 : Inport
  Green_LED : mbd_s32k1xx_ec_toolbox/GPIO Blocks/Digital_Output  gpio_pin=PTD16: [PTD16 | Port D I/O]  init_val=Low  drive_strength=Low
  wires:
  In1/1 -> Green_LED/1

== system flexcan_encrypted_slave_s32k14x/Rx_Complete_Handler/Handle Rx Data/Toggle LEDs/Toggle green LED/Green LED/S32K144 ==
  In1 : Inport
  Green_LED : mbd_s32k1xx_ec_toolbox/GPIO Blocks/Digital_Output  gpio_pin=PTD16: [PTD16 | Port D I/O]  init_val=Low  drive_strength=Low
  Logical Operator : Logic  Operator=NOT  AllPortsSameDT=off  OutDataTypeStr=boolean
  wires:
  In1/1 -> Logical Operator/1
  Logical Operator/1 -> Green_LED/1

== system flexcan_encrypted_slave_s32k14x/Rx_Complete_Handler/Handle Rx Data/Toggle LEDs/Toggle green LED/Green LED/S32K146 ==
  In1 : Inport
  Green_LED : mbd_s32k1xx_ec_toolbox/GPIO Blocks/Digital_Output  gpio_pin=PTD16: [PTD16 | Port D I/O]  init_val=Low  drive_strength=Low
  wires:
  In1/1 -> Green_LED/1

== system flexcan_encrypted_slave_s32k14x/Rx_Complete_Handler/Handle Rx Data/Toggle LEDs/Toggle green LED/Green LED/S32K148 ==
  In1 : Inport
  Green_LED : mbd_s32k1xx_ec_toolbox/GPIO Blocks/Digital_Output  gpio_pin=PTE22: [PTE22 | Port E I/O]  init_val=Low  drive_strength=Low
  wires:
  In1/1 -> Green_LED/1

== system flexcan_encrypted_slave_s32k14x/Rx_Complete_Handler/Handle Rx Data/Toggle LEDs/Toggle red LED/Red LED/S32K142 ==
  In1 : Inport
  Red_LED : mbd_s32k1xx_ec_toolbox/GPIO Blocks/Digital_Output  gpio_pin=PTD15: [PTD15 | Port D I/O]  init_val=Low  drive_strength=Low
  wires:
  In1/1 -> Red_LED/1

== system flexcan_encrypted_slave_s32k14x/Rx_Complete_Handler/Handle Rx Data/Toggle LEDs/Toggle red LED/Red LED/S32K144 ==
  In1 : Inport
  Logical Operator : Logic  Operator=NOT  AllPortsSameDT=off  OutDataTypeStr=boolean
  Red_LED : mbd_s32k1xx_ec_toolbox/GPIO Blocks/Digital_Output  gpio_pin=PTD15: [PTD15 | Port D I/O]  init_val=Low  drive_strength=Low
  wires:
  In1/1 -> Logical Operator/1
  Logical Operator/1 -> Red_LED/1

== system flexcan_encrypted_slave_s32k14x/Rx_Complete_Handler/Handle Rx Data/Toggle LEDs/Toggle red LED/Red LED/S32K146 ==
  In1 : Inport
  Red_LED : mbd_s32k1xx_ec_toolbox/GPIO Blocks/Digital_Output  gpio_pin=PTD15: [PTD15 | Port D I/O]  init_val=Low  drive_strength=Low
  wires:
  In1/1 -> Red_LED/1

== system flexcan_encrypted_slave_s32k14x/Rx_Complete_Handler/Handle Rx Data/Toggle LEDs/Toggle red LED/Red LED/S32K148 ==
  In1 : Inport
  Red_LED : mbd_s32k1xx_ec_toolbox/GPIO Blocks/Digital_Output  gpio_pin=PTE21: [PTE21 | Port E I/O]  init_val=Low  drive_strength=Low
  wires:
  In1/1 -> Red_LED/1

== stateflow chart Rx_Complete_Handler/Handle Rx Data/Toggle LEDs/Toggle green LED/Chart ==
  state A
  state A1
  (default) -> A
  A -> A1
  A1 -> A
  data: A output boolean

== stateflow chart Rx_Complete_Handler/Handle Rx Data/Toggle LEDs/Toggle red LED/Chart ==
  state A
  state A1
  (default) -> A
  A -> A1
  A1 -> A
  data: A output boolean
